simulink model "process"  (R2021a)
settings: Solver=FixedStepDiscrete  StartTime=0.0  StopTime=10  FixedStep=time_step  RelTol=1e-3
model workspace (MAT data in the model file):
  time_step = 0.01
values from neighbouring files (symbols this model uses):
  kGrdCmdSize = uint8(1)    [crc_constants.m]
  kGrdCrcSize = uint8(1)    [crc_constants.m]
  kGrdFrameStart = uint8(hex2dec('0xEF'))    [crc_constants.m]
  kGrdFrameStartSize = uint8(1)    [crc_constants.m]
  kGrdMsgIdSize = uint8(1)    [crc_constants.m]
  kMaxPacketSize = uint8(4)    [crc_constants.m]
undefined symbols (not defined in the file or in its folder): DiscIntNeverNeededParam, Serial_Port, Standard_Devices
libraries: sldrtlib x4
settings Model: OrderedModelArguments=off  Creator=Rahul Subramanian  LastModifiedBy=Rahul Subramanian
settings SolverCC: AlgebraicLoopSolver=TrustRegion
settings DebuggingCC: SFMachineParentedDataDiag=warning
settings RTWCC: Description=Simulink Desktop Real-Time  SystemTargetFile=sldrt.tlc  TemplateMakefile=sldrt.tmf  RTWCompilerOptimization=on
settings CodeAppCC: MaxIdLength=95
settings SimulinkDesktopRealTimeCC: TargetPreCompLibLocation=C:\Program Files\MATLAB\R2021a\toolbox\sldrt\lib\win64

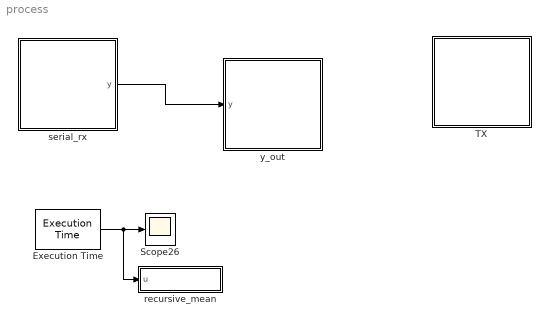
== system process ==
  Execution Time : sldrtlib/Target Profiling/Execution Time  ShowTaskTimes=off
      settings: SourceProductBaseCode=WT
  Scope26 : Scope
  TX : Subsystem
  recursive_mean : Subsystem
  serial_rx : Subsystem
  y_out : Subsystem
  wires:
  Execution Time/1 -> recursive_mean/1(u), Scope26/1
  serial_rx/1(y) -> y_out/1(y)

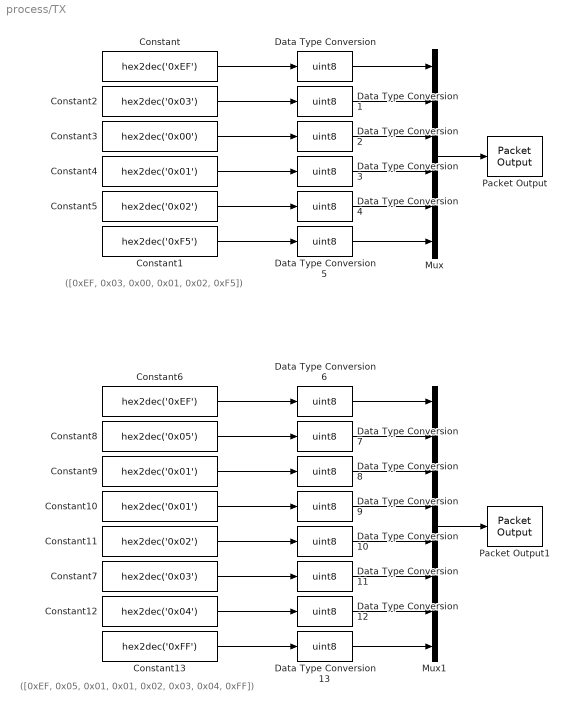
== system process/TX ==
  note: ([0xEF, 0x05, 0x01, 0x01, 0x02, 0x03, 0x04, 0xFF])
  note: ([0xEF, 0x03, 0x00, 0x01, 0x02, 0xF5])
  Constant : Constant  Value=hex2dec('0xEF')
  Constant1 : Constant  Value=hex2dec('0xF5')
  Constant10 : Constant  Value=hex2dec('0x01')
  Constant11 : Constant  Value=hex2dec('0x02')
  Constant12 : Constant  Value=hex2dec('0x04')
  Constant13 : Constant  Value=hex2dec('0xFF')
  Constant2 : Constant  Value=hex2dec('0x03')
  Constant3 : Constant  Value=hex2dec('0x00')
  Constant4 : Constant  Value=hex2dec('0x01')
  Constant5 : Constant  Value=hex2dec('0x02')
  Constant6 : Constant  Value=hex2dec('0xEF')
  Constant7 : Constant  Value=hex2dec('0x03')
  Constant8 : Constant  Value=hex2dec('0x05')
  Constant9 : Constant  Value=hex2dec('0x01')
  Data Type Conversion{,1..13} (14 alike) : DataTypeConversion  OutDataTypeStr=uint8
  Mux : Mux  Inputs=6
  Mux1 : Mux  Inputs=8
  Packet Output : sldrtlib/Packet Output  SampleTime=time_step  MaxMissedTicks=inf  ShowMissedTicks=off  YieldWhenWaiting=off  DrvName=Standard_Devices/Serial_Port  DrvAddress=5  DrvOptions=[115200 8 0 0 0 0 0 0]  PacketSize=6  DataTypes='6*uint8'  ShowReady=off  ShowError=off  PacketID=1  ByteOrder=1  InitialValue=[]  FinalValue=[]
      settings: AttributesFormatString=Serial Port [5]
  Packet Output1 : sldrtlib/Packet Output  SampleTime=time_step  MaxMissedTicks=inf  ShowMissedTicks=off  YieldWhenWaiting=off  DrvName=Standard_Devices/Serial_Port  DrvAddress=5  DrvOptions=[115200 8 0 0 0 0 0 0]  PacketSize=8  DataTypes='8*uint8'  ShowReady=off  ShowError=off  PacketID=1  ByteOrder=1  InitialValue=[]  FinalValue=[]
      settings: AttributesFormatString=Serial Port [5]
  wires:
  Constant3/1 -> Data Type Conversion2/1
  Data Type Conversion5/1 -> Mux/6
  Data Type Conversion1/1 -> Mux/2
  Constant7/1 -> Data Type Conversion11/1
  Constant11/1 -> Data Type Conversion10/1
  Data Type Conversion13/1 -> Mux1/8
  Constant12/1 -> Data Type Conversion12/1
  Data Type Conversion/1 -> Mux/1
  Constant1/1 -> Data Type Conversion5/1
  Mux1/1 -> Packet Output1/1
  Constant2/1 -> Data Type Conversion1/1
  Data Type Conversion8/1 -> Mux1/3
  Constant/1 -> Data Type Conversion/1
  Constant4/1 -> Data Type Conversion3/1
  Data Type Conversion9/1 -> Mux1/4
  Constant5/1 -> Data Type Conversion4/1
  Data Type Conversion3/1 -> Mux/4
  Constant10/1 -> Data Type Conversion9/1
  Mux/1 -> Packet Output/1
  Data Type Conversion4/1 -> Mux/5
  Data Type Conversion2/1 -> Mux/3
  Data Type Conversion11/1 -> Mux1/6
  Data Type Conversion10/1 -> Mux1/5
  Data Type Conversion6/1 -> Mux1/1
  Data Type Conversion7/1 -> Mux1/2
  Constant9/1 -> Data Type Conversion8/1
  Constant8/1 -> Data Type Conversion7/1
  Constant6/1 -> Data Type Conversion6/1
  Data Type Conversion12/1 -> Mux1/7
  Constant13/1 -> Data Type Conversion13/1

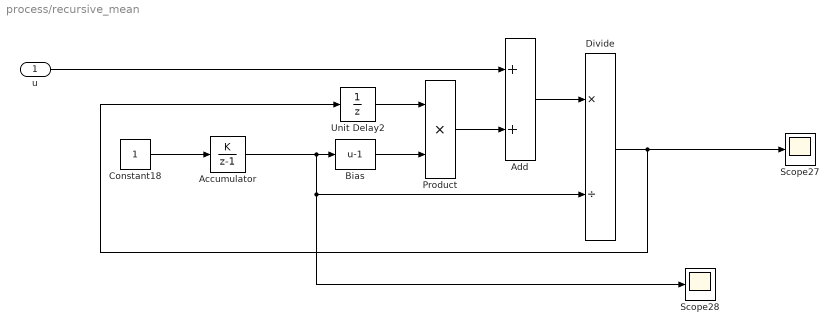
== system process/recursive_mean ==
  u : Inport
  Accumulator : DiscreteIntegrator  IntegratorMethod=Accumulation: Forward Euler  InitialCondition=1  SampleTime=-1  ICPrevOutput=DiscIntNeverNeededParam  ICPrevScaledInput=DiscIntNeverNeededParam
  Add : Sum
  Bias : Bias  Bias=-1
  Constant18 : Constant
  Divide : Product  Inputs=*/
  Product : Product
  Scope27 : Scope
  Scope28 : Scope
  Unit Delay2 : UnitDelay  SampleTime=-1  HasFrameUpgradeWarning=on
  wires:
  Bias/1 -> Product/2
  Constant18/1 -> Accumulator/1
  Accumulator/1 -> Scope28/1, Divide/2, Bias/1
  Add/1 -> Divide/1
  Divide/1 -> Unit Delay2/1, Scope27/1
  Unit Delay2/1 -> Product/1
  Product/1 -> Add/2
  u/1 -> Add/1

== system process/serial_rx ==
  Constant18 : Constant  Value=true
  message_rx_looper : Subsystem  TreatAsAtomicUnit=on
  y : Outport
  wires:
  Constant18/1 -> message_rx_looper/1(whilte_loop_init_cond)
  message_rx_looper/1(y) -> y/1

== system process/y_out ==
  y : Inport
  Display : Display
  wires:
  y/1 -> Display/1

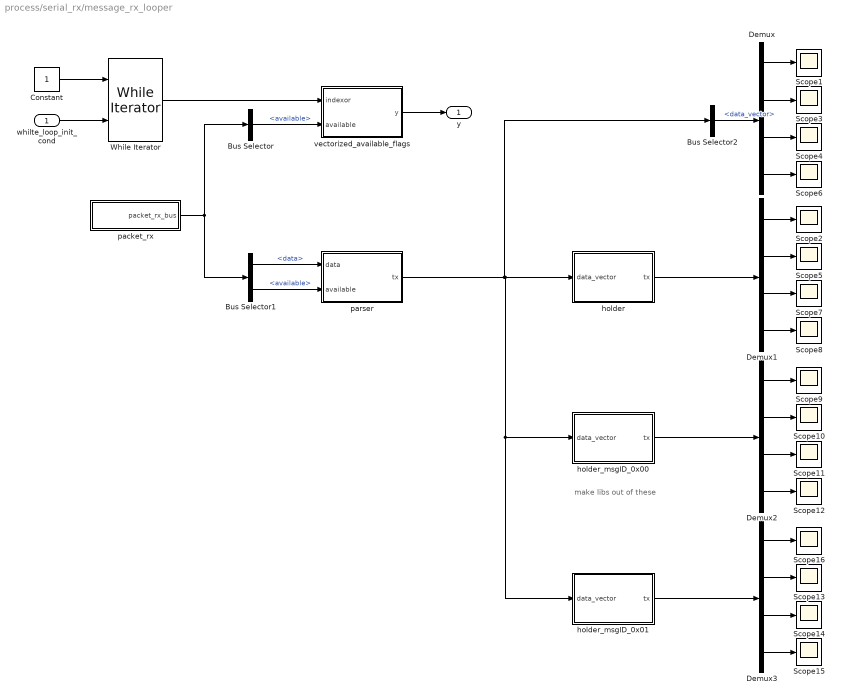
== system process/serial_rx/message_rx_looper ==
  note: make libs out of these
  whilte_loop_init_cond : Inport
  Bus Selector : BusSelector  OutputSignals=available
  Bus Selector1 : BusSelector  OutputSignals=data,available
  Bus Selector2 : BusSelector  OutputSignals=data_vector
  Constant : Constant
  Demux{,1..3} (4 alike) : Demux
  Scope{1..16} (16 alike) : Scope
  While Iterator : WhileIterator  MaxIters=message_poll_num  ShowIterationPort=on  OutputDataType=uint8
  holder : Subsystem
  holder_msgID_0x00 : Subsystem
  holder_msgID_0x01 : Subsystem
  packet_rx : Subsystem
  parser : Subsystem
  vectorized_available_flags : Subsystem
  y : Outport
  wires:
  While Iterator/1 -> vectorized_available_flags/1(indexor)
  whilte_loop_init_cond/1 -> While Iterator/2
  vectorized_available_flags/1(y) -> y/1
  Constant/1 -> While Iterator/1
  packet_rx/1(packet_rx_bus) -> Bus Selector1/1, Bus Selector/1
  Bus Selector/1 -> vectorized_available_flags/2(available)  "<available>"
  Bus Selector1/1 -> parser/1(data)  "<data>"
  Bus Selector1/2 -> parser/2(available)  "<available>"
  Demux/4 -> Scope6/1
  Bus Selector2/1 -> Demux/1  "<data_vector>"
  Demux/2 -> Scope3/1
  Demux/1 -> Scope1/1
  Demux/3 -> Scope4/1
  parser/1(tx) -> holder_msgID_0x01/1(data_vector), holder_msgID_0x00/1(data_vector), holder/1(data_vector), Bus Selector2/1
  holder/1(tx) -> Demux1/1
  Demux1/4 -> Scope8/1
  Demux1/2 -> Scope5/1
  Demux1/1 -> Scope2/1
  Demux1/3 -> Scope7/1
  Demux2/3 -> Scope11/1
  Demux2/1 -> Scope9/1
  Demux2/2 -> Scope10/1
  Demux2/4 -> Scope12/1
  holder_msgID_0x00/1(tx) -> Demux2/1
  holder_msgID_0x01/1(tx) -> Demux3/1
  Demux3/4 -> Scope15/1
  Demux3/2 -> Scope13/1
  Demux3/1 -> Scope16/1
  Demux3/3 -> Scope14/1

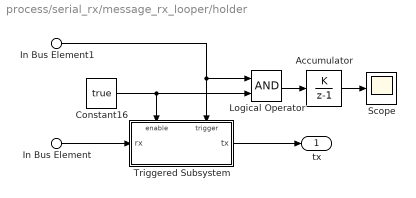
== system process/serial_rx/message_rx_looper/holder ==
  In Bus Element : Inport  PortName=data_vector  Element=data_vector
  In Bus Element1 : Inport  PortName=data_vector  Element=new_data
  Accumulator : DiscreteIntegrator  IntegratorMethod=Accumulation: Forward Euler  SampleTime=-1  OutDataTypeStr=uint16  ICPrevOutput=DiscIntNeverNeededParam  ICPrevScaledInput=DiscIntNeverNeededParam
  Constant16 : Constant  Value=true
  Logical Operator : Logic  AllPortsSameDT=off  OutDataTypeStr=boolean
  Scope : Scope
  Triggered Subsystem : Subsystem  TreatAsAtomicUnit=on
  tx : Outport
  wires:
  Constant16/1 -> Logical Operator/2, Triggered Subsystem/Enable
  In Bus Element/1 -> Triggered Subsystem/1(rx)
  In Bus Element1/1 -> Logical Operator/1, Triggered Subsystem/Trigger
  Triggered Subsystem/1(tx) -> tx/1
  Logical Operator/1 -> Accumulator/1
  Accumulator/1 -> Scope/1

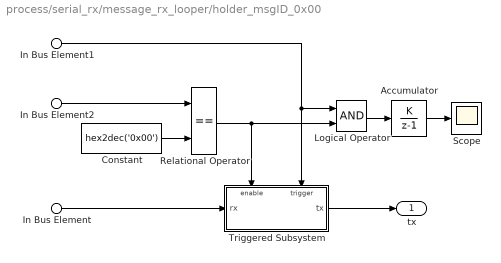
== system process/serial_rx/message_rx_looper/holder_msgID_0x00 ==
  In Bus Element : Inport  PortName=data_vector  Element=data_vector
  In Bus Element1 : Inport  PortName=data_vector  Element=new_data
  In Bus Element2 : Inport  PortName=data_vector  Element=msg_id
  Accumulator : DiscreteIntegrator  IntegratorMethod=Accumulation: Forward Euler  SampleTime=-1  OutDataTypeStr=uint16  ICPrevOutput=DiscIntNeverNeededParam  ICPrevScaledInput=DiscIntNeverNeededParam
  Constant : Constant  Value=hex2dec('0x00')
  Logical Operator : Logic  AllPortsSameDT=off  OutDataTypeStr=boolean
  Relational Operator : RelationalOperator  Operator===  OutDataTypeStr=boolean  RndMeth=Simplest
  Scope : Scope
  Triggered Subsystem : Subsystem  TreatAsAtomicUnit=on
  tx : Outport
  wires:
  Triggered Subsystem/1(tx) -> tx/1
  In Bus Element1/1 -> Logical Operator/1, Triggered Subsystem/Trigger
  In Bus Element/1 -> Triggered Subsystem/1(rx)
  Relational Operator/1 -> Logical Operator/2, Triggered Subsystem/Enable
  In Bus Element2/1 -> Relational Operator/1
  Constant/1 -> Relational Operator/2
  Logical Operator/1 -> Accumulator/1
  Accumulator/1 -> Scope/1

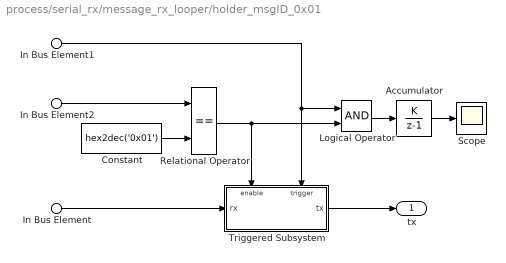
== system process/serial_rx/message_rx_looper/holder_msgID_0x01 ==
  In Bus Element : Inport  PortName=data_vector  Element=data_vector
  In Bus Element1 : Inport  PortName=data_vector  Element=new_data
  In Bus Element2 : Inport  PortName=data_vector  Element=msg_id
  Accumulator : DiscreteIntegrator  IntegratorMethod=Accumulation: Forward Euler  SampleTime=-1  OutDataTypeStr=uint16  ICPrevOutput=DiscIntNeverNeededParam  ICPrevScaledInput=DiscIntNeverNeededParam
  Constant : Constant  Value=hex2dec('0x01')
  Logical Operator : Logic  AllPortsSameDT=off  OutDataTypeStr=boolean
  Relational Operator : RelationalOperator  Operator===  OutDataTypeStr=boolean  RndMeth=Simplest
  Scope : Scope
  Triggered Subsystem : Subsystem  TreatAsAtomicUnit=on
  tx : Outport
  wires:
  Constant/1 -> Relational Operator/2
  In Bus Element2/1 -> Relational Operator/1
  Relational Operator/1 -> Logical Operator/2, Triggered Subsystem/Enable
  In Bus Element/1 -> Triggered Subsystem/1(rx)
  In Bus Element1/1 -> Logical Operator/1, Triggered Subsystem/Trigger
  Triggered Subsystem/1(tx) -> tx/1
  Logical Operator/1 -> Accumulator/1
  Accumulator/1 -> Scope/1

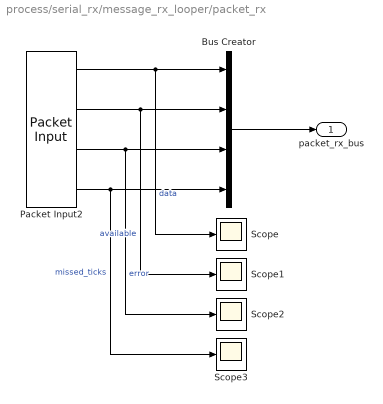
== system process/serial_rx/message_rx_looper/packet_rx ==
  Bus Creator : BusCreator  Inputs=4
  Packet Input2 : sldrtlib/Packet Input  SampleTime=-1  MaxMissedTicks=inf  ShowMissedTicks=on  YieldWhenWaiting=off  DrvName=Standard_Devices/Serial_Port  DrvAddress=5  DrvOptions=[115200 8 0 0 0 0 0 0]  PacketSize=1  DataTypes='1*uint8'  ShowReady=on  ShowError=on  PacketID=1  ByteOrder=1  ShowTimestamp=off
      settings: AttributesFormatString=Serial Port [5]
  Scope{,1..3} (4 alike) : Scope
  packet_rx_bus : Outport
  wires:
  Packet Input2/4 -> Bus Creator/4, Scope3/1  "missed_ticks"
  Packet Input2/1 -> Bus Creator/1, Scope/1  "data"
  Packet Input2/2 -> Bus Creator/2, Scope1/1  "available"
  Packet Input2/3 -> Bus Creator/3, Scope2/1  "error"
  Bus Creator/1 -> packet_rx_bus/1

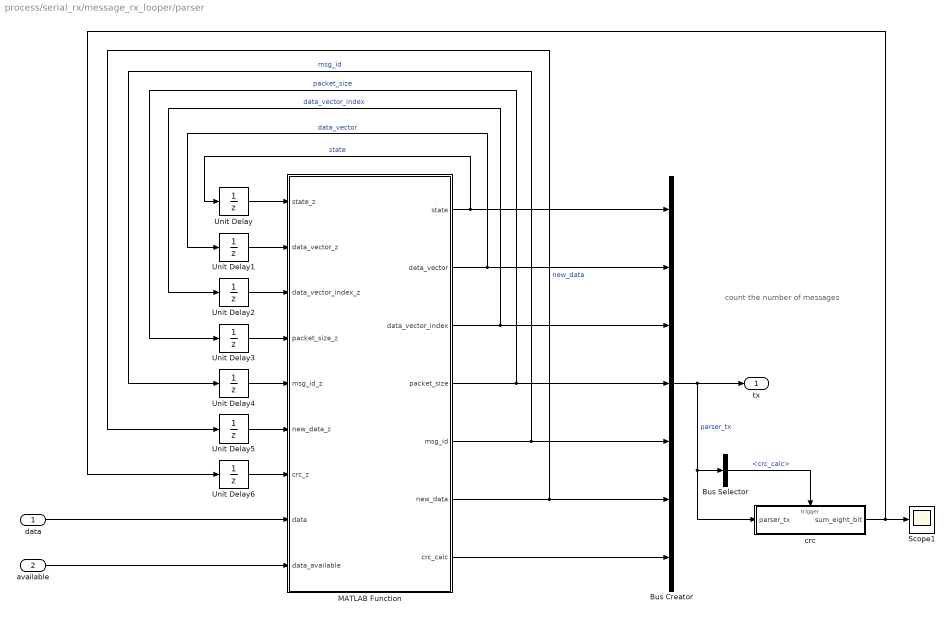
== system process/serial_rx/message_rx_looper/parser ==
  note: count the number of messages
  data : Inport
  available : Inport  Port=2
  Bus Creator : BusCreator  Inputs=7
  Bus Selector : BusSelector  OutputSignals=crc_calc
  MATLAB Function : MATLAB Function  TreatAsAtomicUnit=on
  Scope1 : Scope
  Unit Delay : UnitDelay  InitialCondition=uint8(1)  SampleTime=-1  HasFrameUpgradeWarning=on
  Unit Delay1 : UnitDelay  SampleTime=-1  HasFrameUpgradeWarning=on
  Unit Delay2 : UnitDelay  InitialCondition=1  SampleTime=-1  HasFrameUpgradeWarning=on
  Unit Delay3 : UnitDelay  SampleTime=-1  HasFrameUpgradeWarning=on
  Unit Delay4 : UnitDelay  SampleTime=-1  HasFrameUpgradeWarning=on
  Unit Delay5 : UnitDelay  InitialCondition=false  SampleTime=-1  HasFrameUpgradeWarning=on
  Unit Delay6 : UnitDelay  InitialCondition=uint8(0)  SampleTime=-1  HasFrameUpgradeWarning=on
  crc : Subsystem
  tx : Outport
  wires:
  data/1 -> MATLAB Function/8(data)
  MATLAB Function/1(state) -> Unit Delay/1, Bus Creator/1  "state"
  Unit Delay/1 -> MATLAB Function/1(state_z)
  Unit Delay3/1 -> MATLAB Function/4(packet_size_z)
  MATLAB Function/2(data_vector) -> Unit Delay1/1, Bus Creator/2  "data_vector"
  Unit Delay1/1 -> MATLAB Function/2(data_vector_z)
  MATLAB Function/5(msg_id) -> Unit Delay4/1, Bus Creator/5  "msg_id"
  available/1 -> MATLAB Function/9(data_available)
  MATLAB Function/4(packet_size) -> Unit Delay3/1, Bus Creator/4  "packet_size"
  MATLAB Function/3(data_vector_index) -> Unit Delay2/1, Bus Creator/3  "data_vector_index"
  Unit Delay2/1 -> MATLAB Function/3(data_vector_index_z)
  Unit Delay4/1 -> MATLAB Function/5(msg_id_z)
  Unit Delay5/1 -> MATLAB Function/6(new_data_z)
  MATLAB Function/6(new_data) -> Bus Creator/6, Unit Delay5/1  "new_data"
  Bus Creator/1 -> Bus Selector/1, crc/1(parser_tx), tx/1  "parser_tx"
  Unit Delay6/1 -> MATLAB Function/7(crc_z)
  crc/1(sum_eight_bit) -> Unit Delay6/1, Scope1/1
  Bus Selector/1 -> crc/Trigger  "<crc_calc>"
  MATLAB Function/7(crc_calc) -> Bus Creator/7

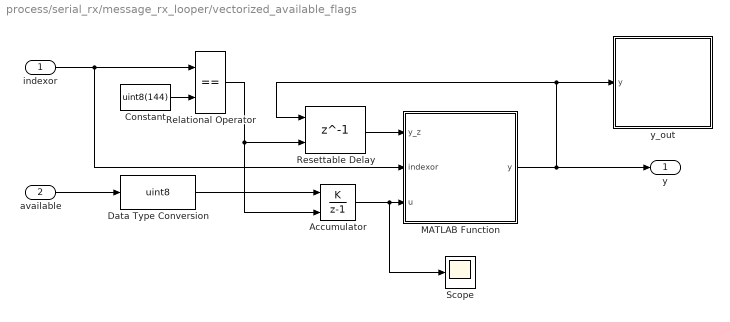
== system process/serial_rx/message_rx_looper/vectorized_available_flags ==
  indexor : Inport
  available : Inport  Port=2
  Accumulator : DiscreteIntegrator  IntegratorMethod=Accumulation: Forward Euler  ExternalReset=level  SampleTime=-1  ICPrevOutput=DiscIntNeverNeededParam  ICPrevScaledInput=DiscIntNeverNeededParam
  Constant : Constant  Value=uint8(144)
  Data Type Conversion : DataTypeConversion  OutDataTypeStr=uint8
  MATLAB Function : MATLAB Function  TreatAsAtomicUnit=on
  Relational Operator : RelationalOperator  Operator===  OutDataTypeStr=boolean  RndMeth=Simplest
  Resettable Delay : Delay  DelayLength=1  ExternalReset=Falling
      settings: InputPortMap=u0,r5
  Scope : Scope
  y_out : Subsystem
  y : Outport
  wires:
  Data Type Conversion/1 -> Accumulator/1
  MATLAB Function/1(y) -> y_out/1(y), Resettable Delay/1, y/1
  Accumulator/1 -> Scope/1, MATLAB Function/3(u)
  Resettable Delay/1 -> MATLAB Function/1(y_z)
  available/1 -> Data Type Conversion/1
  indexor/1 -> MATLAB Function/2(indexor), Relational Operator/1
  Constant/1 -> Relational Operator/2
  Relational Operator/1 -> Resettable Delay/2, Accumulator/2

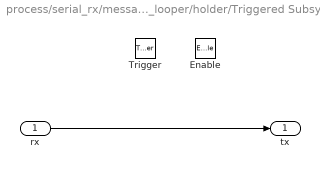
== system process/serial_rx/message_rx_looper/holder/Triggered Subsystem ==
  rx : Inport
  Enable : EnablePort
  Trigger : TriggerPort  VariantControl=(inherit)
  tx : Outport
  wires:
  rx/1 -> tx/1

== system process/serial_rx/message_rx_looper/holder_msgID_0x00/Triggered Subsystem ==
  rx : Inport
  Enable : EnablePort
  Trigger : TriggerPort  VariantControl=(inherit)
  tx : Outport
  wires:
  rx/1 -> tx/1

== system process/serial_rx/message_rx_looper/holder_msgID_0x01/Triggered Subsystem ==
  rx : Inport
  Enable : EnablePort
  Trigger : TriggerPort  VariantControl=(inherit)
  tx : Outport
  wires:
  rx/1 -> tx/1

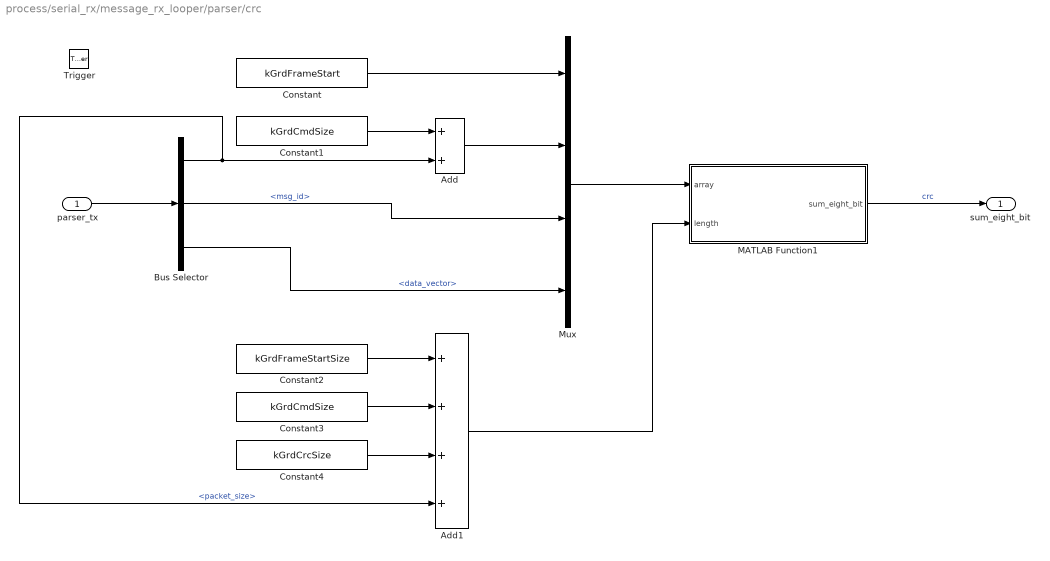
== system process/serial_rx/message_rx_looper/parser/crc ==
  parser_tx : Inport
  Trigger : TriggerPort  VariantControl=(inherit)  PortDimensions=1
  Add : Sum
  Add1 : Sum  Inputs=4
  Bus Selector : BusSelector  OutputSignals=packet_size,msg_id,data_vector
  Constant : Constant  Value=kGrdFrameStart
  Constant1 : Constant  Value=kGrdCmdSize
  Constant2 : Constant  Value=kGrdFrameStartSize
  Constant3 : Constant  Value=kGrdCmdSize
  Constant4 : Constant  Value=kGrdCrcSize
  MATLAB Function1 : MATLAB Function  TreatAsAtomicUnit=on
  Mux : Mux
  sum_eight_bit : Outport
  wires:
  Mux/1 -> MATLAB Function1/1(array)
  Constant2/1 -> Add1/1
  Constant1/1 -> Add/1
  MATLAB Function1/1(sum_eight_bit) -> sum_eight_bit/1  "crc"
  Add/1 -> Mux/2
  Bus Selector/1 -> Add/2, Add1/4  "<packet_size>"
  Constant3/1 -> Add1/2
  Constant/1 -> Mux/1
  Bus Selector/2 -> Mux/3  "<msg_id>"
  Constant4/1 -> Add1/3
  Bus Selector/3 -> Mux/4  "<data_vector>"
  parser_tx/1 -> Bus Selector/1
  Add1/1 -> MATLAB Function1/2(length)

== system process/serial_rx/message_rx_looper/vectorized_available_flags/y_out ==
  y : Inport
  Display : Display
  wires:
  y/1 -> Display/1

== matlab function process/serial_rx/message_rx_looper/parser/crc/MATLAB Function1 ==
  data: array input; sum_eight_bit output; length input
function sum_eight_bit = ComputeCRC(array, length) 

sum = uint16(0);

for j = 1:length
    sum = sum + uint16(array(j));
end
if (sum > hex2dec('0xFF'))
    sum = bitshift(sum, -8) + bitand(sum, hex2dec('0xFF'));
end

sum_eight_bit = uint8(sum);

end

== matlab function process/serial_rx/message_rx_looper/parser/MATLAB Function ==
  data: state_z input uint8; data_vector_z input uint8 size=4; data_vector_index_z input uint8; packet_size_z input uint8; msg_id_z input uint8; new_data_z input boolean; crc_z input uint8; data input uint8; state output uint8; data_available input boolean; data_vector output uint8 size=4; data_vector_index output uint8; packet_size output uint8; msg_id output uint8; new_data output boolean; kGrdFrameStart parameter; kMaxPacketSize parameter; kGrdFrameStartSize parameter; kGrdCmdSize parameter; kGrdMsgIdSize parameter; kGrdCrcSize parameter; crc_calc output
function [state, data_vector, data_vector_index, packet_size, msg_id, new_data, crc_calc] = fcn(state_z, data_vector_z, data_vector_index_z, packet_size_z, msg_id_z, new_data_z, crc_z, data, data_available, kGrdFrameStart, kMaxPacketSize, kGrdFrameStartSize, kGrdCmdSize, kGrdMsgIdSize, kGrdCrcSize)

% Description:
% 1. Reads each byte, finds a header and then creates a new data flag.
% 2. Data can be read from data_vector
% 3. Constants have been defined outside this program

% temp
% crc = uint8(0);
crc_calc = false;

% read previous state
state = state_z;
data_vector = data_vector_z;
data_vector_index = data_vector_index_z;
packet_size = packet_size_z;
msg_id = msg_id_z;
new_data = new_data_z;
crc = crc_z;

% switch on state.
% state is used to indicate which stage of the data packet read the parser
% is in
switch state
    
    case uint8(1)
        % reset variable states for new message
        new_data = false;
        msg_id = uint8(0);
        data_vector = uint8(zeros(4,1));
        data_vector_index = uint8(1);
        packet_size = uint8(0);
        crc = uint8(0);
        if data_available % if new data byte is available
            if data == kGrdFrameStart % if this is a header
                state = state + 1; % iterate state
            end
        end

    case uint8(2)
        if data_available % if new data byte is available
            packet_size = data - kGrdCmdSize; % this is the packet payload size
            state = state + 1; % iterate state
        end

    case uint8(3)
        if data_available % if new data byte is available
            msg_id = data; % store the message ID
            state = state + 1; % iterate state
        end

    case uint8(4)
        if data_available % if new data byte is available
            data_vector(data_vector_index) = data; % grab data in a vector
            
            if data_vector_index == packet_size % if packet_size is reached
                state = state + 1; % iterate state
                % calculate the crc here
                crc_calc = true; % trigger crc calc
            end
            
            data_vector_index = data_vector_index + 1; % iterate indexor for each byte stored

        end

	case uint8(5) % for grabbing the crc
        crc_calc = false;
        if data_available % if new data byte is available
            if crc == data
                new_data = true; % call the function
                state = uint8(1);
                
            end
        end
end % end of switch case

end

== matlab function process/serial_rx/message_rx_looper/vectorized_available_flags/MATLAB Function ==
  data: y_z input; indexor input; u input uint8; y output uint8 size=144
function y = fcn(y_z, indexor, u)

y = y_z;
y(indexor) = u;
